simulink model "sistema"  (R2022b)
settings: Solver=VariableStepAuto  StartTime=0.0  StopTime=200  RelTol=1e-3
undefined symbols (not defined in the file or in its folder): Kp_PID, Kp_PID_2, Td_2, Td_PID, Ti_PID, Ti_PID_2
settings Model: Creator=heloi  LastModifiedBy=heloi

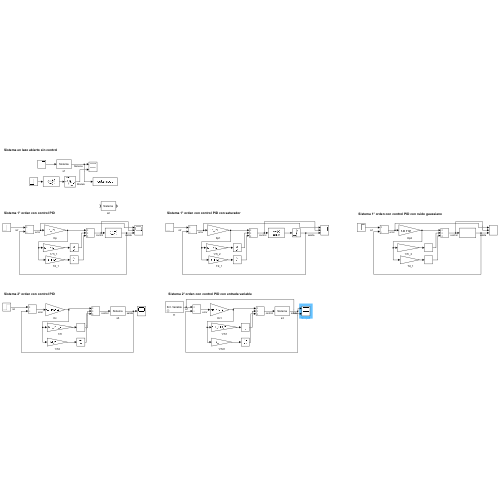
[thumbnail: Simulink's stored preview of the top-level diagram]
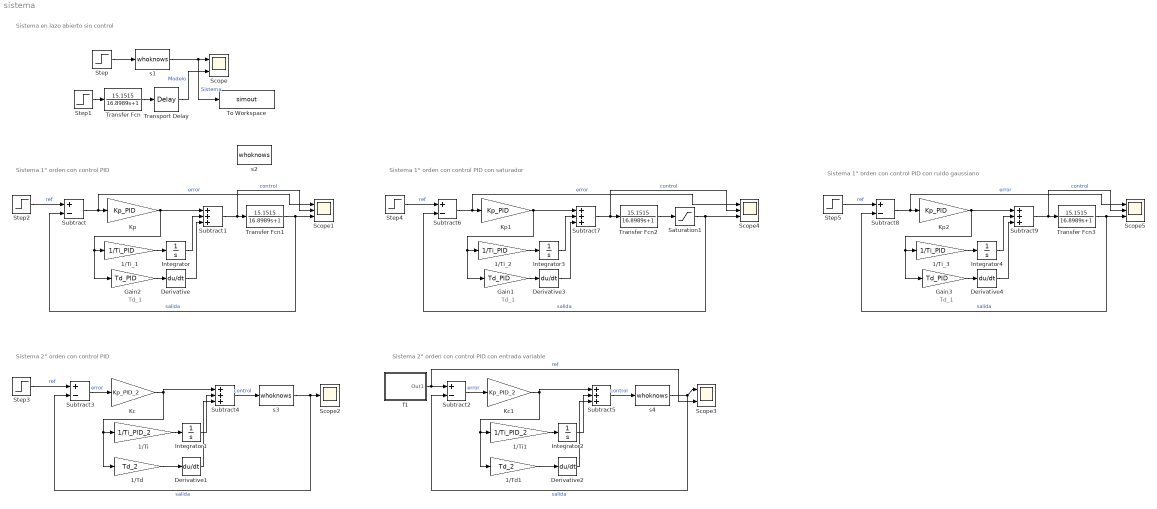
== system sistema ==
  note: Td_1
  note: Sistema 1° orden con control PID
  note: Sistema en lazo abierto sin control
  note: Sistema 2° orden con control PID
  note: Sistema 2° orden con control PID con entrada variable
  note: Td_1
  note: Sistema 1° orden con control PID con saturador
  note: Td_1
  note: Sistema 1° orden con control PID con ruido gaussiano
  1/Td : Gain  Gain=Td_2
  1/Td1 : Gain  Gain=Td_2
  1/Ti : Gain  Gain=1/Ti_PID_2
  1/Ti1 : Gain  Gain=1/Ti_PID_2
  1/Ti_1 : Gain  Gain=1/Ti_PID
  1/Ti_2 : Gain  Gain=1/Ti_PID
  1/Ti_3 : Gain  Gain=1/Ti_PID
  Derivative{,1..4} (5 alike) : Derivative
  Gain1 : Gain  Gain=Td_PID
  Gain2 : Gain  Gain=Td_PID
  Gain3 : Gain  Gain=Td_PID
  Integrator{,1..4} (5 alike) : Integrator
  Kc : Gain  Gain=Kp_PID_2
  Kc1 : Gain  Gain=Kp_PID_2
  Kp : Gain  Gain=Kp_PID
  Kp1 : Gain  Gain=Kp_PID
  Kp2 : Gain  Gain=Kp_PID
  Saturation1 : Saturate  UpperLimit=1  LowerLimit=-1
  Scope : Scope  NumInputPorts=2
  Scope1 : Scope  NumInputPorts=3
  Scope2 : Scope
  Scope3 : Scope  NumInputPorts=2
  Scope4 : Scope  NumInputPorts=3
  Scope5 : Scope  NumInputPorts=3
  Step{,1..5} (6 alike) : Step  SampleTime=0
  Subtract{,2..3,6,8} (5 alike) : Sum  Inputs=+-
  Subtract{1,4..5,7,9} (5 alike) : Sum  Inputs=+++
  To Workspace : ToWorkspace  VariableName=simout  SaveFormat=Timeseries  SampleTime=-1
  Transfer Fcn{,1..3} (4 alike) : TransferFcn  Numerator=15.1515  Denominator=[16.8989 1]
  Transport Delay : TransportDelay  DelayTime=1.25
  f1 : Subsystem  mask{S=1, L=0, T=2}
      mask prompts: S "Limite Superior"; L "Limite Inferior"; T "Periodo de cambio"
      mask Display: disp('Ent. Variable')
  s1 : M-S-Function  FunctionName=whoknows  Parameters=L, P1, P2, T, R  mask{L=6, P1=0, P2=9, T=1, R=0}
      mask prompts: L "Laboratorio"; P1 "Primer digito del Puesto"; P2 "Segundo digito del Puesto"; T "Tipo de Planta"; R "Ruido"
      mask Display: disp('Sistema')
  s2 : M-S-Function  FunctionName=whoknows  Parameters=L, P1, P2, T, R  mask{L=6, P1=0, P2=9, T=1, R=0}
      mask prompts: L "Laboratorio"; P1 "Primer digito del Puesto"; P2 "Segundo digito del Puesto"; T "Tipo de Planta"; R "Ruido"
      mask Display: disp('Sistema')
  s3 : M-S-Function  FunctionName=whoknows  Parameters=L, P1, P2, T, R  mask{L=6, P1=0, P2=9, T=2, R=0}
      mask prompts: L "Laboratorio"; P1 "Primer digito del Puesto"; P2 "Segundo digito del Puesto"; T "Tipo de Planta"; R "Ruido"
      mask Display: disp('Sistema')
  s4 : M-S-Function  FunctionName=whoknows  Parameters=L, P1, P2, T, R  mask{L=6, P1=0, P2=9, T=2, R=0}
      mask prompts: L "Laboratorio"; P1 "Primer digito del Puesto"; P2 "Segundo digito del Puesto"; T "Tipo de Planta"; R "Ruido"
      mask Display: disp('Sistema')
  wires:
  s1/1 -> To Workspace/1, Scope/1  "Sistema"
  Step/1 -> s1/1
  Transfer Fcn/1 -> Transport Delay/1
  Step1/1 -> Transfer Fcn/1
  Step2/1 -> Subtract/1  "ref"
  Subtract/1 -> Scope1/1, Kp/1  "error"
  Transport Delay/1 -> Scope/2  "Modelo"
  Kp/1 -> Subtract1/1, Gain2/1, 1/Ti_1/1
  s3/1 -> Scope2/1, Subtract3/2  "salida"
  Step3/1 -> Subtract3/1  "ref"
  Subtract3/1 -> Kc/1  "error"
  Kc/1 -> 1/Td/1, 1/Ti/1, Subtract4/1
  Subtract4/1 -> s3/1  "control"
  1/Td/1 -> Derivative1/1
  1/Ti/1 -> Integrator1/1
  Integrator1/1 -> Subtract4/2
  Derivative1/1 -> Subtract4/3
  1/Ti_1/1 -> Integrator/1
  Gain2/1 -> Derivative/1
  Integrator/1 -> Subtract1/2
  Derivative/1 -> Subtract1/3
  Subtract1/1 -> Transfer Fcn1/1, Scope1/2  "control"
  Subtract5/1 -> s4/1  "control"
  Derivative2/1 -> Subtract5/3
  1/Ti1/1 -> Integrator2/1
  f1/1(Out1) -> Scope3/2, Subtract2/1  "ref"
  Kc1/1 -> 1/Td1/1, 1/Ti1/1, Subtract5/1
  1/Td1/1 -> Derivative2/1
  s4/1 -> Scope3/1, Subtract2/2  "salida"
  Integrator2/1 -> Subtract5/2
  Subtract2/1 -> Kc1/1  "error"
  Transfer Fcn1/1 -> Scope1/3, Subtract/2  "salida"
  Saturation1/1 -> Subtract6/2, Scope4/3  "salida"
  Subtract7/1 -> Transfer Fcn2/1, Scope4/2  "control"
  Transfer Fcn2/1 -> Saturation1/1
  Derivative3/1 -> Subtract7/3
  1/Ti_2/1 -> Integrator3/1
  Integrator3/1 -> Subtract7/2
  Step4/1 -> Subtract6/1  "ref"
  Kp1/1 -> Subtract7/1, Gain1/1, 1/Ti_2/1
  Subtract6/1 -> Scope4/1, Kp1/1  "error"
  Gain1/1 -> Derivative3/1
  Transfer Fcn3/1 -> Scope5/3, Subtract8/2  "salida"
  Subtract9/1 -> Transfer Fcn3/1, Scope5/2  "control"
  Derivative4/1 -> Subtract9/3
  1/Ti_3/1 -> Integrator4/1
  Integrator4/1 -> Subtract9/2
  Step5/1 -> Subtract8/1  "ref"
  Kp2/1 -> Subtract9/1, Gain3/1, 1/Ti_3/1
  Subtract8/1 -> Scope5/1, Kp2/1  "error"
  Gain3/1 -> Derivative4/1

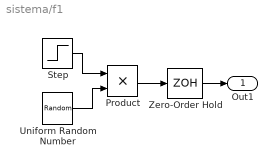
== system sistema/f1 ==
  Product : Product  RndMeth=Zero
  Step : Step  Time=0  SampleTime=0
  Uniform Random Number : UniformRandomNumber  Minimum=L  Maximum=S  SampleTime=0
  Zero-Order Hold : ZeroOrderHold  SampleTime=T
  Out1 : Outport
  wires:
  Step/1 -> Product/1
  Uniform Random Number/1 -> Product/2
  Product/1 -> Zero-Order Hold/1
  Zero-Order Hold/1 -> Out1/1
